simulink model "Two_area_system_with_wind_farm-DESKTOP-8DA4B7M"  (R2020a)
settings: Solver=ode23tb  StartTime=0.0  StopTime=20  RelTol=1e-3
InitFcn:
  | initAll
values from neighbouring files (symbols this model uses):
  DCgridinit = nDCgrid_init(resultsdc,wB)    [initAll.m]
  Geninit = Generator_init(opdata,SynMach_in_gidx)    [initAll.m]
  SdcgridB = resultsdc.baseMVAdc    [initAll.m]
  SgridB = resultsac.baseMVA    [initAll.m]
  VSCinit = converter_init(resultsac,resultsdc)    [initAll.m]
  wB = 2*pi*fB    (= 314.159265359)    [initAll.m]
undefined symbols (not defined in the file or in its folder): ACgirdinit, AVm0, c1, c2, c3, c4, c5, c6, cp_nom, lambda_nom, P_wind_base, Pelec_base, Pnom, Windinit
libraries: powerlib_meascontrol x9, simulink_extras x1
(part 1 of 4)
settings Model: Creator=LinSiQi  LastModifiedBy=Qiufan_Yang
settings DataIOCC: SaveOutput=off  SignalLogging=off  DSMLogging=off  SaveTime=off  ReturnWorkspaceOutputs=off
settings DebuggingCC: ArithmeticOperatorsInVariantConditions=warning
settings SFSimCC: CustomCodeUndefinedFunction=UseInterfaceOnly
settings CodeAppCC: StateflowObjectComments=on
settings SimscapeCC: SimscapeNormalizeSystem=off

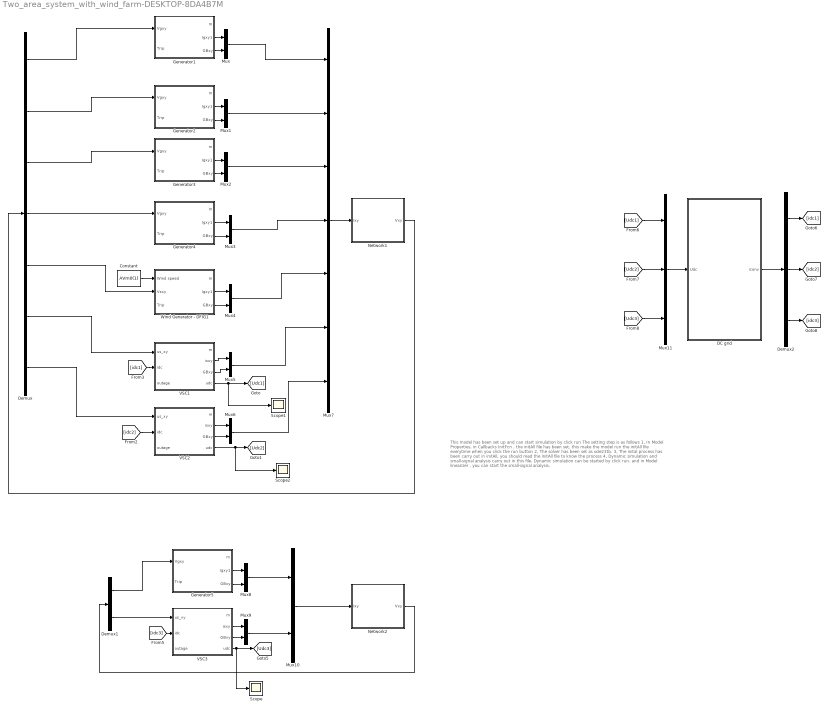
== system Two_area_system_with_wind_farm-DESKTOP-8DA4B7M ==
  note: This model has been set up and can start simulation by click run
      |
      | The setting step is as follows
      | 1, In Model Properties, in Callbacks InitFcn , the initAll file has been set, this make the model run the initAll file everytime when you click the run button
      |
      | 2, The solver has been set as ode23tb.
      |
      | 3, The inital process has been carry out in initAll, you should read the initAll file to know the process
      |
      | 4, Dynamic simulation and small-signal analysis carry out in this file. Dynamic simulation can be started by click run. and in Model linearizer , you can start the small-signal analysis.
  Constant : Constant  Value=AVm0(1)
  DC grid : Subsystem  mask{Rdc=DCgridinit.RdcA, Ldc=DCgridinit.LdcA, TDC=DCgridinit.TDC, TDCt=DCgridinit.TDCt, Idc=DCgridinit.IdcA}
  Demux : Demux  Outputs=7
  Demux1 : Demux  Outputs=2
  Demux2 : Demux  Outputs=3
  Generator1 : Subsystem  mask{wB=wB, SgenB=Geninit.SgenB(1), SgridB=SgridB, Xq=Geninit.Xq(1), Xq1=Geninit.Xq1(1), Xq11=Geninit.Xq11(1), Tq0=Geninit.Tq0(1), Tq10=Geninit.Tq10(1), Eq10=Geninit.Eq1(1), Eq110=Geninit.Eq11(1), Xd=Geninit.Xd(1), Xd1=Geninit.Xd1(1), Xd11=Geninit.Xd11(1), Td0=Geninit.Td0(1), Td10=Geninit.Td10(1), Ed10=Geninit.Ed1(1), Ed110=Geninit.Ed11(1), H=Geninit.Tj(1), D=Geninit.D(1), delta0=Geninit.Delta(1), w0=1, Pm0=Geninit.Pm0(1), Ka=Geninit.Ka(1), Tb=Geninit.Tb(1), Tc=Geninit.Tc(1), Efmin=Geninit.Efmin(1), Efmax=Geninit.Efmax(1), Vref=Geninit.Vref(1), Ef10=Geninit.Vf1(1), S_PSS=Geninit.EnablePSS(1), Kpss=Geninit.kpss(1), Tw_P=Geninit.Tw_P(1), T1_P=Geninit.T1_P(1), T2_P=Geninit.T2_P(1), T3_P=Geninit.T3_P(1), T4_P=Geninit.T4_P(1), Upmax=Geninit.Upmax(1), Upmin=Geninit.Upmin(1), S_Gov=Geninit.Enablegov(1), R=Geninit.R_G(1), Ts_G=Geninit.Ts_G(1), Tc_G=Geninit.Tc_G(1), T3_G=Geninit.T3_G(1), T4_G=Geninit.T4_G(1), T5_G=Geninit.T5_G(1), dPmax=Geninit.dPmax(1), dPmin=Geninit.dPmin(1)}
      mask prompts: S_PSS "Enable PSS"; Tw_P "Tw"; T1_P "T1"; T2_P "T2"; T3_P "T3"; T4_P "T4"; S_Gov "Enable Governor"; Ts_G "Ts"; Tc_G "Tc"; T3_G "T3"; T4_G "T4"; T5_G "T5"
      mask help: This is a six-order synchronous generator with exciter system, governor and PSS.
      mask DialogControl Container6 Prompt: Machine parameter
      mask DialogControl Container25 Prompt: Base value
      mask DialogControl Container3 Prompt: q axis parameter
      mask DialogControl ParameterGroupVar Prompt: d axis parameter
      mask DialogControl Container4 Prompt: machine parameter
      mask DialogControl Container12 Prompt: Excitation System parameter
      mask DialogControl Container22 Prompt: parameter
      mask DialogControl Container23 Prompt: inital value
      mask DialogControl Container10 Prompt: PSS parameter
      mask DialogControl Container13 Prompt: Governor parameter
  Generator2 : Subsystem  mask{wB=wB, SgenB=Geninit.SgenB(2), SgridB=SgridB, Xq=Geninit.Xq(2), Xq1=Geninit.Xq1(2), Xq11=Geninit.Xq11(2), Tq0=Geninit.Tq0(2), Tq10=Geninit.Tq10(2), Eq10=Geninit.Eq1(2), Eq110=Geninit.Eq11(2), Xd=Geninit.Xd(2), Xd1=Geninit.Xd1(2), Xd11=Geninit.Xd11(2), Td0=Geninit.Td0(2), Td10=Geninit.Td10(2), Ed10=Geninit.Ed1(2), Ed110=Geninit.Ed11(2), H=Geninit.Tj(2), D=Geninit.D(2), delta0=Geninit.Delta(2), w0=1, Pm0=Geninit.Pm0(2), Ka=Geninit.Ka(2), Tb=Geninit.Tb(2), Tc=Geninit.Tc(2), Efmin=Geninit.Efmin(2), Efmax=Geninit.Efmax(2), Vref=Geninit.Vref(2), Ef10=Geninit.Vf1(2), S_PSS=Geninit.EnablePSS(2), Kpss=Geninit.kpss(2), Tw_P=Geninit.Tw_P(2), T1_P=Geninit.T1_P(2), T2_P=Geninit.T2_P(2), T3_P=Geninit.T3_P(2), T4_P=Geninit.T4_P(2), Upmax=Geninit.Upmax(2), Upmin=Geninit.Upmin(2), S_Gov=Geninit.Enablegov(2), R=Geninit.R_G(2), Ts_G=Geninit.Ts_G(2), Tc_G=Geninit.Tc_G(2), T3_G=Geninit.T3_G(2), T4_G=Geninit.T4_G(2), T5_G=Geninit.T5_G(2), dPmax=Geninit.dPmax(2), dPmin=Geninit.dPmin(2)}
      mask prompts: S_PSS "Enable PSS"; Tw_P "Tw"; T1_P "T1"; T2_P "T2"; T3_P "T3"; T4_P "T4"; S_Gov "Enable Governor"; Ts_G "Ts"; Tc_G "Tc"; T3_G "T3"; T4_G "T4"; T5_G "T5"
      mask help: This is a six-order synchronous generator with exciter system, governor and PSS.
      mask DialogControl Container6 Prompt: Machine parameter
      mask DialogControl Container25 Prompt: Base value
      mask DialogControl Container3 Prompt: q axis parameter
      mask DialogControl ParameterGroupVar Prompt: d axis parameter
      mask DialogControl Container4 Prompt: machine parameter
      mask DialogControl Container12 Prompt: Excitation System parameter
      mask DialogControl Container22 Prompt: parameter
      mask DialogControl Container23 Prompt: inital value
      mask DialogControl Container10 Prompt: PSS parameter
      mask DialogControl Container13 Prompt: Governor parameter
  Generator3 : Subsystem  mask{wB=wB, SgenB=Geninit.SgenB(3), SgridB=SgridB, Xq=Geninit.Xq(3), Xq1=Geninit.Xq1(3), Xq11=Geninit.Xq11(3), Tq0=Geninit.Tq0(3), Tq10=Geninit.Tq10(3), Eq10=Geninit.Eq1(3), Eq110=Geninit.Eq11(3), Xd=Geninit.Xd(3), Xd1=Geninit.Xd1(3), Xd11=Geninit.Xd11(3), Td0=Geninit.Td0(3), Td10=Geninit.Td10(3), Ed10=Geninit.Ed1(3), Ed110=Geninit.Ed11(3), H=Geninit.Tj(3), D=Geninit.D(3), delta0=Geninit.Delta(3), w0=1, Pm0=Geninit.Pm0(3), Ka=Geninit.Ka(3), Tb=Geninit.Tb(3), Tc=Geninit.Tc(3), Efmin=Geninit.Efmin(3), Efmax=Geninit.Efmax(3), Vref=Geninit.Vref(3), Ef10=Geninit.Vf1(3), S_PSS=Geninit.EnablePSS(3), Kpss=Geninit.kpss(3), Tw_P=Geninit.Tw_P(3), T1_P=Geninit.T1_P(3), T2_P=Geninit.T2_P(3), T3_P=Geninit.T3_P(3), T4_P=Geninit.T4_P(3), Upmax=Geninit.Upmax(3), Upmin=Geninit.Upmin(3), S_Gov=Geninit.Enablegov(3), R=Geninit.R_G(3), Ts_G=Geninit.Ts_G(3), Tc_G=Geninit.Tc_G(3), T3_G=Geninit.T3_G(3), T4_G=Geninit.T4_G(3), T5_G=Geninit.T5_G(3), dPmax=Geninit.dPmax(3), dPmin=Geninit.dPmin(3)}
      mask prompts: S_PSS "Enable PSS"; Tw_P "Tw"; T1_P "T1"; T2_P "T2"; T3_P "T3"; T4_P "T4"; S_Gov "Enable Governor"; Ts_G "Ts"; Tc_G "Tc"; T3_G "T3"; T4_G "T4"; T5_G "T5"
      mask help: This is a six-order synchronous generator with exciter system, governor and PSS.
      mask DialogControl Container6 Prompt: Machine parameter
      mask DialogControl Container25 Prompt: Base value
      mask DialogControl Container3 Prompt: q axis parameter
      mask DialogControl ParameterGroupVar Prompt: d axis parameter
      mask DialogControl Container4 Prompt: machine parameter
      mask DialogControl Container12 Prompt: Excitation System parameter
      mask DialogControl Container22 Prompt: parameter
      mask DialogControl Container23 Prompt: inital value
      mask DialogControl Container10 Prompt: PSS parameter
      mask DialogControl Container13 Prompt: Governor parameter
  Generator4 : Subsystem  mask{wB=wB, SgenB=Geninit.SgenB(4), SgridB=SgridB, Xq=Geninit.Xq(4), Xq1=Geninit.Xq1(4), Xq11=Geninit.Xq11(4), Tq0=Geninit.Tq0(4), Tq10=Geninit.Tq10(4), Eq10=Geninit.Eq1(4), Eq110=Geninit.Eq11(4), Xd=Geninit.Xd(4), Xd1=Geninit.Xd1(4), Xd11=Geninit.Xd11(4), Td0=Geninit.Td0(4), Td10=Geninit.Td10(4), Ed10=Geninit.Ed1(4), Ed110=Geninit.Ed11(4), H=Geninit.Tj(4), D=Geninit.D(4), delta0=Geninit.Delta(4), w0=1, Pm0=Geninit.Pm0(4), Ka=Geninit.Ka(4), Tb=Geninit.Tb(4), Tc=Geninit.Tc(4), Efmin=Geninit.Efmin(4), Efmax=Geninit.Efmax(4), Vref=Geninit.Vref(4), Ef10=Geninit.Vf1(4), S_PSS=Geninit.EnablePSS(4), Kpss=Geninit.kpss(4), Tw_P=Geninit.Tw_P(4), T1_P=Geninit.T1_P(4), T2_P=Geninit.T2_P(4), T3_P=Geninit.T3_P(4), T4_P=Geninit.T4_P(4), Upmax=Geninit.Upmax(4), Upmin=Geninit.Upmin(4), S_Gov=Geninit.Enablegov(4), R=Geninit.R_G(4), Ts_G=Geninit.Ts_G(4), Tc_G=Geninit.Tc_G(4), T3_G=Geninit.T3_G(4), T4_G=Geninit.T4_G(4), T5_G=Geninit.T5_G(4), dPmax=Geninit.dPmax(4), dPmin=Geninit.dPmin(4)}
      mask prompts: S_PSS "Enable PSS"; Tw_P "Tw"; T1_P "T1"; T2_P "T2"; T3_P "T3"; T4_P "T4"; S_Gov "Enable Governor"; Ts_G "Ts"; Tc_G "Tc"; T3_G "T3"; T4_G "T4"; T5_G "T5"
      mask help: This is a six-order synchronous generator with exciter system, governor and PSS.
      mask DialogControl Container6 Prompt: Machine parameter
      mask DialogControl Container25 Prompt: Base value
      mask DialogControl Container3 Prompt: q axis parameter
      mask DialogControl ParameterGroupVar Prompt: d axis parameter
      mask DialogControl Container4 Prompt: machine parameter
      mask DialogControl Container12 Prompt: Excitation System parameter
      mask DialogControl Container22 Prompt: parameter
      mask DialogControl Container23 Prompt: inital value
      mask DialogControl Container10 Prompt: PSS parameter
      mask DialogControl Container13 Prompt: Governor parameter
  Generator5 : Subsystem  mask{wB=wB, SgenB=Geninit.SgenB(5), SgridB=SgridB, Xq=Geninit.Xq(5), Xq1=Geninit.Xq1(5), Xq11=Geninit.Xq11(5), Tq0=Geninit.Tq0(5), Tq10=Geninit.Tq10(5), Eq10=Geninit.Eq1(5), Eq110=Geninit.Eq11(5), Xd=Geninit.Xd(5), Xd1=Geninit.Xd1(5), Xd11=Geninit.Xd11(5), Td0=Geninit.Td0(5), Td10=Geninit.Td10(5), Ed10=Geninit.Ed1(5), Ed110=Geninit.Ed11(5), H=Geninit.Tj(5), D=Geninit.D(5), delta0=Geninit.Delta(5), w0=1, Pm0=Geninit.Pm0(5), Ka=Geninit.Ka(5), Tb=Geninit.Tb(5), Tc=Geninit.Tc(5), Efmin=Geninit.Efmin(5), Efmax=Geninit.Efmax(5), Vref=Geninit.Vref(5), Ef10=Geninit.Vf1(5), S_PSS=Geninit.EnablePSS(5), Kpss=Geninit.kpss(5), Tw_P=Geninit.Tw_P(5), T1_P=Geninit.T1_P(5), T2_P=Geninit.T2_P(5), T3_P=Geninit.T3_P(5), T4_P=Geninit.T4_P(5), Upmax=Geninit.Upmax(5), Upmin=Geninit.Upmin(5), S_Gov=Geninit.Enablegov(5), R=Geninit.R_G(5), Ts_G=Geninit.Ts_G(5), Tc_G=Geninit.Tc_G(5), T3_G=Geninit.T3_G(5), T4_G=Geninit.T4_G(5), T5_G=Geninit.T5_G(5), dPmax=Geninit.dPmax(5), dPmin=Geninit.dPmin(5)}
      mask prompts: S_PSS "Enable PSS"; Tw_P "Tw"; T1_P "T1"; T2_P "T2"; T3_P "T3"; T4_P "T4"; S_Gov "Enable Governor"; Ts_G "Ts"; Tc_G "Tc"; T3_G "T3"; T4_G "T4"; T5_G "T5"
      mask help: This is a six-order synchronous generator with exciter system, governor and PSS.
      mask DialogControl Container6 Prompt: Machine parameter
      mask DialogControl Container25 Prompt: Base value
      mask DialogControl Container3 Prompt: q axis parameter
      mask DialogControl ParameterGroupVar Prompt: d axis parameter
      mask DialogControl Container4 Prompt: machine parameter
      mask DialogControl Container12 Prompt: Excitation System parameter
      mask DialogControl Container22 Prompt: parameter
      mask DialogControl Container23 Prompt: inital value
      mask DialogControl Container10 Prompt: PSS parameter
      mask DialogControl Container13 Prompt: Governor parameter
  Mux{,1..6,8..10} (10 alike) : Mux  Inputs=2
  Mux11 : Mux  Inputs=3
  Mux7 : Mux  Inputs=7
  Network1 : Subsystem  mask{busdata=ACgirdinit.busdata{1}, linedata=ACgirdinit.linedata{1}, VSS0=ACgirdinit.VSS0{1}, LINE=ACgirdinit.fline{1}, fbus=ACgirdinit.FBUS(1), ng=ACgirdinit.ng{1}, Currentin_idx=ACgirdinit.Currentin_idx{1}}
  Network2 : Subsystem  mask{busdata=ACgirdinit.busdata{2}, linedata=ACgirdinit.linedata{2}, VSS0=ACgirdinit.VSS0{2}, LINE=ACgirdinit.fline{2}, fbus=ACgirdinit.FBUS(2), ng=ACgirdinit.ng{2}, Currentin_idx=ACgirdinit.Currentin_idx{2}}
  Scope : Scope
  Scope1 : Scope
  Scope2 : Scope
  VSC1 : Subsystem  mask{Vdcbase=VSCinit.Vdcbase(1), Vnom=VSCinit.Vacbase(1), SvscB=VSCinit.SvscBi(1), SgridB=SgridB, SdcgridB=SdcgridB, Kppll_VSC=VSCinit.Kppll(1), Kipll_VSC=VSCinit.Kipll(1), Dels_hvdc=VSCinit.Dels_hvdc(1), CeqA=VSCinit.CeqA(1), UeqA=VSCinit.UeqA(1), Lpr=VSCinit.Lpr(1), Rpr=VSCinit.Rpr(1), wB=wB, Is_xA_0=VSCinit.Isx0(1), Is_yA_0=VSCinit.Isy0(1), d_axis_control=VSCinit.d_axis_control(1), KpP_VSC_A=VSCinit.KpP(1), KiP_VSC_A=VSCinit.KiP(1), Kpdc_VSC_A=VSCinit.Kpdc(1), Kidc_VSC_A=VSCinit.Kidc(1), KpId_VSC_A=VSCinit.KpId(1), KiId_VSC_A=VSCinit.KiId(1), q_axis_control=VSCinit.q_axis_control(1), KpQ_VSC_A=VSCinit.KpQ(1), KiQ_VSC_A=VSCinit.KiQ(1), Kpac_VSC_A=VSCinit.Kpac(1), Kiac_VSC_A=VSCinit.Kiac(1), KpIq_VSC_A=VSCinit.KpIq(1), KiIq_VSC_A=VSCinit.KiIq(1), Md_A_0=VSCinit.Md0(1), Mq_A_0=VSCinit.Mq0(1), Nd_A_0=VSCinit.Nd0(1), Nq_A_0=VSCinit.Nq0(1), Pref=VSCinit.Pref(1), Udcref=VSCinit.Udcref(1), Qref=VSCinit.Qref(1), Uref=VSCinit.Uref(1)}
      mask prompts: Vnom "Vacbase"; Kppll_VSC "Kppll"; Kipll_VSC "Kipll"; KpP_VSC_A "KpP"; KiP_VSC_A "KiP"; Kpdc_VSC_A "Kpdc"; Kidc_VSC_A "Kidc"; KpId_VSC_A "KpId"; KiId_VSC_A "KiId"; KpQ_VSC_A "KpQ"; KiQ_VSC_A "KiQ"; Kpac_VSC_A "Kpac"; Kiac_VSC_A "Kiac"; KpIq_VSC_A "KpIq"; KiIq_VSC_A "KiIq"
      mask DialogControl Container48 Prompt: Base value
      mask DialogControl Container7 Prompt: PLL
      mask DialogControl Container5 Prompt: Control parameter
      mask DialogControl Container8 Prompt: inital value
      mask DialogControl Container12 Prompt: DC side
      mask DialogControl Container13 Prompt: Parameter
      mask DialogControl Container15 Prompt: Initial value
      mask DialogControl Container9 Prompt: AC side
      mask DialogControl Container10 Prompt: Parameter
      mask DialogControl Container11 Prompt: Initial value
      mask DialogControl Container18 Prompt: Control parameter
      mask DialogControl Container19 Prompt: d_axis_control parameter
      mask DialogControl Container23 Prompt: d_axis_control=1
      mask DialogControl Container24 Prompt: d_axis_control=2
      mask DialogControl Container26 Prompt: inner current control
      mask DialogControl Container21 Prompt: q_axis_control parameter
      mask DialogControl Container29 Prompt: q_axis_control=1
      mask DialogControl Container30 Prompt: q_axis_control=2
      mask DialogControl Container31 Prompt: inner current control
      mask DialogControl Container22 Prompt: inital value
      mask DialogControl Container35 Prompt: outer controller
      mask DialogControl Container36 Prompt: inner control
      mask DialogControl Container38 Prompt: Reference
  VSC2 : Subsystem  mask{Vdcbase=VSCinit.Vdcbase(2), Vnom=VSCinit.Vacbase(2), SvscB=VSCinit.SvscBi(2), SgridB=SgridB, SdcgridB=SdcgridB, Kppll_VSC=VSCinit.Kppll(2), Kipll_VSC=VSCinit.Kipll(2), Dels_hvdc=VSCinit.Dels_hvdc(2), CeqA=VSCinit.CeqA(2), UeqA=VSCinit.UeqA(2), Lpr=VSCinit.Lpr(2), Rpr=VSCinit.Rpr(2), wB=wB, Is_xA_0=VSCinit.Isx0(2), Is_yA_0=VSCinit.Isy0(2), d_axis_control=VSCinit.d_axis_control(2), KpP_VSC_A=VSCinit.KpP(2), KiP_VSC_A=VSCinit.KiP(2), Kpdc_VSC_A=VSCinit.Kpdc(2), Kidc_VSC_A=VSCinit.Kidc(2), KpId_VSC_A=VSCinit.KpId(2), KiId_VSC_A=VSCinit.KiId(2), q_axis_control=VSCinit.q_axis_control(2), KpQ_VSC_A=VSCinit.KpQ(2), KiQ_VSC_A=VSCinit.KiQ(2), Kpac_VSC_A=VSCinit.Kpac(2), Kiac_VSC_A=VSCinit.Kiac(2), KpIq_VSC_A=VSCinit.KpIq(2), KiIq_VSC_A=VSCinit.KiIq(2), Md_A_0=VSCinit.Md0(2), Mq_A_0=VSCinit.Mq0(2), Nd_A_0=VSCinit.Nd0(2), Nq_A_0=VSCinit.Nq0(2), Pref=VSCinit.Pref(2), Udcref=VSCinit.Udcref(2), Qref=VSCinit.Qref(2), Uref=VSCinit.Uref(2)}
      mask prompts: Vnom "Vacbase"; Kppll_VSC "Kppll"; Kipll_VSC "Kipll"; KpP_VSC_A "KpP"; KiP_VSC_A "KiP"; Kpdc_VSC_A "Kpdc"; Kidc_VSC_A "Kidc"; KpId_VSC_A "KpId"; KiId_VSC_A "KiId"; KpQ_VSC_A "KpQ"; KiQ_VSC_A "KiQ"; Kpac_VSC_A "Kpac"; Kiac_VSC_A "Kiac"; KpIq_VSC_A "KpIq"; KiIq_VSC_A "KiIq"
      mask DialogControl Container48 Prompt: Base value
      mask DialogControl Container7 Prompt: PLL
      mask DialogControl Container5 Prompt: Control parameter
      mask DialogControl Container8 Prompt: inital value
      mask DialogControl Container12 Prompt: DC side
      mask DialogControl Container13 Prompt: Parameter
      mask DialogControl Container15 Prompt: Initial value
      mask DialogControl Container9 Prompt: AC side
      mask DialogControl Container10 Prompt: Parameter
      mask DialogControl Container11 Prompt: Initial value
      mask DialogControl Container18 Prompt: Control parameter
      mask DialogControl Container19 Prompt: d_axis_control parameter
      mask DialogControl Container23 Prompt: d_axis_control=1
      mask DialogControl Container24 Prompt: d_axis_control=2
      mask DialogControl Container26 Prompt: inner current control
      mask DialogControl Container21 Prompt: q_axis_control parameter
      mask DialogControl Container29 Prompt: q_axis_control=1
      mask DialogControl Container30 Prompt: q_axis_control=2
      mask DialogControl Container31 Prompt: inner current control
      mask DialogControl Container22 Prompt: inital value
      mask DialogControl Container35 Prompt: outer controller
      mask DialogControl Container36 Prompt: inner control
      mask DialogControl Container38 Prompt: Reference
  VSC3 : Subsystem  mask{Vdcbase=VSCinit.Vdcbase(3), Vnom=VSCinit.Vacbase(3), SvscB=VSCinit.SvscBi(3), SgridB=SgridB, SdcgridB=SdcgridB, Kppll_VSC=VSCinit.Kppll(3), Kipll_VSC=VSCinit.Kipll(3), Dels_hvdc=VSCinit.Dels_hvdc(3), CeqA=VSCinit.CeqA(3), UeqA=VSCinit.UeqA(3), Lpr=VSCinit.Lpr(3), Rpr=VSCinit.Rpr(3), wB=wB, Is_xA_0=VSCinit.Isx0(3), Is_yA_0=VSCinit.Isy0(3), d_axis_control=VSCinit.d_axis_control(3), KpP_VSC_A=VSCinit.KpP(3), KiP_VSC_A=VSCinit.KiP(3), Kpdc_VSC_A=VSCinit.Kpdc(3), Kidc_VSC_A=VSCinit.Kidc(3), KpId_VSC_A=VSCinit.KpId(3), KiId_VSC_A=VSCinit.KiId(3), q_axis_control=VSCinit.q_axis_control(3), KpQ_VSC_A=VSCinit.KpQ(3), KiQ_VSC_A=VSCinit.KiQ(3), Kpac_VSC_A=VSCinit.Kpac(3), Kiac_VSC_A=VSCinit.Kiac(3), KpIq_VSC_A=VSCinit.KpIq(3), KiIq_VSC_A=VSCinit.KiIq(3), Md_A_0=VSCinit.Md0(3), Mq_A_0=VSCinit.Mq0(3), Nd_A_0=VSCinit.Nd0(3), Nq_A_0=VSCinit.Nq0(3), Pref=VSCinit.Pref(3), Udcref=VSCinit.Udcref(3), Qref=VSCinit.Qref(3), Uref=VSCinit.Uref(3)}
      mask prompts: Vnom "Vacbase"; Kppll_VSC "Kppll"; Kipll_VSC "Kipll"; KpP_VSC_A "KpP"; KiP_VSC_A "KiP"; Kpdc_VSC_A "Kpdc"; Kidc_VSC_A "Kidc"; KpId_VSC_A "KpId"; KiId_VSC_A "KiId"; KpQ_VSC_A "KpQ"; KiQ_VSC_A "KiQ"; Kpac_VSC_A "Kpac"; Kiac_VSC_A "Kiac"; KpIq_VSC_A "KpIq"; KiIq_VSC_A "KiIq"
      mask DialogControl Container48 Prompt: Base value
      mask DialogControl Container7 Prompt: PLL
      mask DialogControl Container5 Prompt: Control parameter
      mask DialogControl Container8 Prompt: inital value
      mask DialogControl Container12 Prompt: DC side
      mask DialogControl Container13 Prompt: Parameter
      mask DialogControl Container15 Prompt: Initial value
      mask DialogControl Container9 Prompt: AC side
      mask DialogControl Container10 Prompt: Parameter
      mask DialogControl Container11 Prompt: Initial value
      mask DialogControl Container18 Prompt: Control parameter
      mask DialogControl Container19 Prompt: d_axis_control parameter
      mask DialogControl Container23 Prompt: d_axis_control=1
      mask DialogControl Container24 Prompt: d_axis_control=2
      mask DialogControl Container26 Prompt: inner current control
      mask DialogControl Container21 Prompt: q_axis_control parameter
      mask DialogControl Container29 Prompt: q_axis_control=1
      mask DialogControl Container30 Prompt: q_axis_control=2
      mask DialogControl Container31 Prompt: inner current control
      mask DialogControl Container22 Prompt: inital value
      mask DialogControl Container35 Prompt: outer controller
      mask DialogControl Container36 Prompt: inner control
      mask DialogControl Container38 Prompt: Reference
  Wind Generator - DFIG1 : Subsystem  mask{NN=Windinit.NN(1), SwgBi=Windinit.SwgBi(1), SmecBi=100, SgridB=SgridB, Atheta=Windinit.Atheta(1), Kppll=Windinit.Kppll_wind(1), Kipll=Windinit.Kipll_wind(1), pitch=[500 45 2], Srotors=1.3, H=Windinit.H(1), Wr0=Windinit.Wr0(1), Xa=Windinit.Xa(1), Xa1=Windinit.Xa1(1), Lm=Windinit.Lm(1), Lr=Windinit.Lr(1), Rs=Windinit.Rs(1), Ls=Windinit.Ls(1), Ta0=Windinit.Ta0(1), NPf=Windinit.NPf(1), Za=Windinit.Za{1}, Ex0=Windinit.Ex_ref(1), Ey0=Windinit.Ey_ref(1), wB=wB, KpP_rw=Windinit.KpP_rw(1), KiP_rw=Windinit.KiP_rw(1), KpId_rw=Windinit.KpId_rw(1), KiId_rw=Windinit.KiId_rw(1), KpQ_rw=Windinit.KpQ_rw(1), KiQ_rw=Windinit.KiQ_rw(1), KpIq_rw=Windinit.KpIq_rw(1), KiIq_rw=Windinit.KiIq_rw(1), Ird_ref=Windinit.Ird_ref(1), Irq_ref=Windinit.Irq_ref(1), Qs0=Windinit.Qs0(1), KpDC_gw=Windinit.KpDC_gw(1), KiDC_gw=Windinit.KiDC_gw(1), KpId_gw=Windinit.KpId_gw(1), KiId_gw=Windinit.KiId_gw(1), KpIq_gw=Windinit.KpIq_gw(1), KiIq_gw=Windinit.KiIq_gw(1), Vdc_w=Windinit.Vdc_w(1), Icd_ref=Windinit.Icd_ref(1), Icq_ref=Windinit.Icq_ref(1), Vcd_ref=Windinit.Vcd_ref(1), Vcq_ref=Windinit.Vcq_ref(1), Lg=Windinit.Lg(1), Rg=Windinit.Rg(1), Icx0=Windinit.Icx0(1), Icy0=Windinit.Icy0(1), C_w=Windinit.C_w(1), Vdc0=Windinit.Vdc0(1)}
      mask prompts: pitch "pitch_gain，pitch_max，pitch_rate"; Srotors "Start Rotor Speed"; Ex0 "Ex"; Ey0 "Ey"
      mask init:
      | pitch_gain=pitch(1);
      | pitch_max=pitch(2);
      | pitch_rate=pitch(3);
      | 
      | %该风机模型的基准容量
      | 
      | SwgeqB=SwgBi.*NN;
      mask DialogControl Container4 Prompt: PLL/Wind turbine
      mask DialogControl Container31 Prompt: Base value
      mask DialogControl Container23 Prompt: PLL
      mask DialogControl Container6 Prompt: inital value
      mask DialogControl Container5 Prompt: PI parameter
      mask DialogControl Container24 Prompt: Wind turbine
      mask DialogControl Container25 Prompt: pitch control
      mask DialogControl Container7 Prompt: Machine parameter
      mask DialogControl Container8 Prompt: Rotor
      mask DialogControl Container9 Prompt: Machine
      mask DialogControl Container10 Prompt: parameter
      mask DialogControl Container11 Prompt: inital value
      mask DialogControl Container12 Prompt: Rotor side control
      mask DialogControl Container13 Prompt: Control parameter
      mask DialogControl Container14 Prompt: Initial value
      mask DialogControl Container15 Prompt: reactive power
      mask DialogControl Container16 Prompt: Grid side control
      mask DialogControl Container17 Prompt: parameter
      mask DialogControl Container18 Prompt: reference
      mask DialogControl Container19 Prompt: inital value
      mask DialogControl Container20 Prompt: converter function
      mask DialogControl Container21 Prompt: inital value
      mask DialogControl Container22 Prompt: DC function
  wires:
  Generator1/2(Igxy1) -> Mux/1
  Generator1/3(GBxy) -> Mux/2
  Generator2/2(Igxy1) -> Mux1/1
  Generator2/3(GBxy) -> Mux1/2
  Generator3/2(Igxy1) -> Mux2/1
  Generator3/3(GBxy) -> Mux2/2
  Generator4/2(Igxy1) -> Mux3/1
  Generator4/3(GBxy) -> Mux3/2
  Wind Generator - DFIG1/2(Igxy1) -> Mux4/1
  Wind Generator - DFIG1/3(GBxy) -> Mux4/2
  VSC1/2(isxy) -> Mux5/1
  VSC1/3(GBxy) -> Mux5/2
  VSC2/2(isxy) -> Mux6/1
  VSC2/3(GBxy) -> Mux6/2
  Mux7/1 -> Network1/1(Ixy)
  Mux/1 -> Mux7/1
  Mux1/1 -> Mux7/2
  Mux2/1 -> Mux7/3
  Mux3/1 -> Mux7/4
  Mux4/1 -> Mux7/5
  Mux5/1 -> Mux7/6
  Mux6/1 -> Mux7/7
  Network1/1(Vxy) -> Demux/1
  Demux/1 -> Generator1/1(Vgxy)
  Demux/2 -> Generator2/1(Vgxy)
  Demux/3 -> Generator3/1(Vgxy)
  Demux/4 -> Generator4/1(Vgxy)
  Demux/5 -> Wind Generator - DFIG1/2(Vsxy)
  Demux/6 -> VSC1/1(us_xy)
  Demux/7 -> VSC2/1(us_xy)
  Constant/1 -> Wind Generator - DFIG1/1(Wind speed)
  VSC1/4(udc) -> Scope1/1, [Udc1]
  VSC2/4(udc) -> Scope2/1, [Udc2]
  [idc2] -> VSC2/2(idc)
  [idc1] -> VSC1/2(idc)
  Generator5/2(Igxy1) -> Mux8/1
  Generator5/3(GBxy) -> Mux8/2
  VSC3/2(isxy) -> Mux9/1
  VSC3/3(GBxy) -> Mux9/2
  Mux9/1 -> Mux10/2
  Mux8/1 -> Mux10/1
  Mux10/1 -> Network2/1(Ixy)
  Demux1/1 -> Generator5/1(Vgxy)
  Demux1/2 -> VSC3/1(us_xy)
  [idc3] -> VSC3/2(idc)
  VSC3/4(udc) -> Scope/1, [Udc3]
  Network2/1(Vxy) -> Demux1/1
  [Udc1] -> Mux11/1
  [Udc2] -> Mux11/2
  [Udc3] -> Mux11/3
  Mux11/1 -> DC grid/1(Udc)
  DC grid/1(iconv) -> Demux2/1
  Demux2/1 -> [idc1]
  Demux2/2 -> [idc2]
  Demux2/3 -> [idc3]

== system Two_area_system_with_wind_farm-DESKTOP-8DA4B7M/DC grid ==
  Udc : Inport
  Gain : Gain  Gain=TDCt  Multiplication=Matrix(K*u) (u vector)
  Gain1 : Gain  Gain=TDC  Multiplication=Matrix(K*u) (u vector)
  Idc_line : Integrator  InitialCondition=Idc
  K6 : Gain  Gain=Ldc  SaturateOnIntegerOverflow=on  OutDataTypeStr=Inherit: Same as input  ParamDataTypeStr=Inherit: Same as input
  K7 : Gain  Gain=Rdc  SaturateOnIntegerOverflow=on  OutDataTypeStr=Inherit: Same as input  ParamDataTypeStr=Inherit: Same as input
  Sum1 : Sum  Inputs=|+-  SaturateOnIntegerOverflow=on
  iconv : Outport
  wires:
  K6/1 -> Idc_line/1
  Idc_line/1 -> Gain1/1, K7/1
  Sum1/1 -> K6/1
  K7/1 -> Sum1/2
  Udc/1 -> Gain/1
  Gain/1 -> Sum1/1
  Gain1/1 -> iconv/1

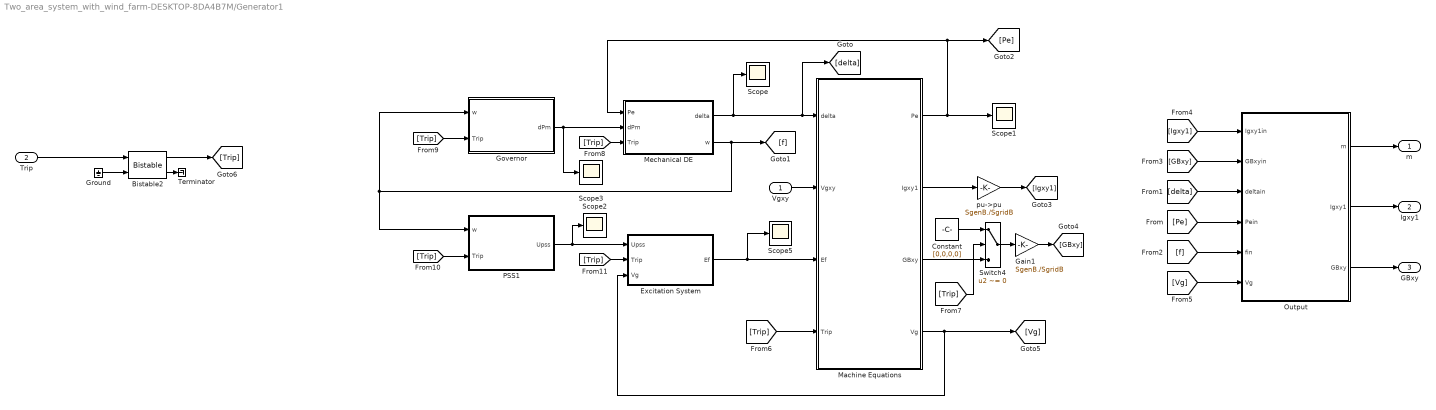
== system Two_area_system_with_wind_farm-DESKTOP-8DA4B7M/Generator1 ==
  Vgxy : Inport
  Trip : Inport  Port=2
  Bistable2 : powerlib_meascontrol/Logic/Bistable  Qpriority=Set  ic=0  Ts=0
      settings: SourceProductBaseCode=PS
  Constant : Constant  Value=[0,0,0,0]
  Excitation System : Subsystem
  Gain1 : Gain  Gain=SgenB./SgridB
  Governor : Subsystem
  Ground : Ground
  "Machine Equations " : Subsystem
  Mechanical DE : Subsystem
  Output : Subsystem
  PSS1 : Subsystem
  Scope{,1..3,5} (5 alike) : Scope
  Switch4 : Switch  Criteria=u2 ~= 0  Threshold=0.5  SaturateOnIntegerOverflow=on
  Terminator : Terminator
  pu->pu : Gain  Gain=SgenB./SgridB
  m : Outport
  Igxy1 : Outport  Port=2
  GBxy : Outport  Port=3
  wires:
  Gain1/1 -> [GBxy]
  pu->pu/1 -> [Igxy1]
  [Trip] -> PSS1/2(Trip)
  [Trip] -> Governor/2(Trip)
  [GBxy] -> Output/2(GBxyin)
  [Trip] -> Excitation System/2(Trip)
  Output/1(m) -> m/1
  Mechanical DE/1(delta) -> Scope/1, "Machine Equations "/1(delta), [delta]
  Bistable2/2 -> Terminator/1
  [f] -> Output/5(fin)
  Output/2(Igxy1) -> Igxy1/1
  PSS1/1(Upss) -> Excitation System/1(Upss), Scope2/1
  "Machine Equations "/3(GBxy) -> Switch4/3
  Vgxy/1 -> "Machine Equations "/2(Vgxy)
  Constant/1 -> Switch4/1
  "Machine Equations "/2(Igxy1) -> pu->pu/1
  Governor/1(dPm) -> Mechanical DE/2(dPm), Scope3/1
  [delta] -> Output/3(deltain)
  [Vg] -> Output/6(Vg)
  [Igxy1] -> Output/1(Igxy1in)
  Mechanical DE/2(w) -> Governor/1(w), PSS1/1(w), [f]
  Output/3(GBxy) -> GBxy/1
  Excitation System/1(Ef) -> Scope5/1, "Machine Equations "/3(Ef)
  "Machine Equations "/4(Vg) -> [Vg], Excitation System/3(Vg)
  [Trip] -> "Machine Equations "/4(Trip)
  [Trip] -> Switch4/2
  Bistable2/1 -> [Trip]
  "Machine Equations "/1(Pe) -> Scope1/1, Mechanical DE/1(Pe), [Pe]
  [Pe] -> Output/4(Pein)
  Switch4/1 -> Gain1/1
  Trip/1 -> Bistable2/1
  Ground/1 -> Bistable2/2
  [Trip] -> Mechanical DE/3(Trip)

== system Two_area_system_with_wind_farm-DESKTOP-8DA4B7M/Generator2 ==
  Vgxy : Inport
  Trip : Inport  Port=2
  Bistable2 : powerlib_meascontrol/Logic/Bistable  Qpriority=Set  ic=0  Ts=0
      settings: SourceProductBaseCode=PS
  Constant : Constant  Value=[0,0,0,0]
  Excitation System : Subsystem
  Gain1 : Gain  Gain=SgenB./SgridB
  Governor : Subsystem
  Ground : Ground
  "Machine Equations " : Subsystem
  Mechanical DE : Subsystem
  Output : Subsystem
  PSS1 : Subsystem
  Scope{,1..3,5} (5 alike) : Scope
  Switch4 : Switch  Criteria=u2 ~= 0  Threshold=0.5  SaturateOnIntegerOverflow=on
  Terminator : Terminator
  pu->pu : Gain  Gain=SgenB./SgridB
  m : Outport
  Igxy1 : Outport  Port=2
  GBxy : Outport  Port=3
  wires:
  Gain1/1 -> [GBxy]
  pu->pu/1 -> [Igxy1]
  [Trip] -> PSS1/2(Trip)
  [Trip] -> Governor/2(Trip)
  [GBxy] -> Output/2(GBxyin)
  [Trip] -> Excitation System/2(Trip)
  Output/1(m) -> m/1
  Mechanical DE/1(delta) -> Scope/1, "Machine Equations "/1(delta), [delta]
  Bistable2/2 -> Terminator/1
  [f] -> Output/5(fin)
  Output/2(Igxy1) -> Igxy1/1
  PSS1/1(Upss) -> Excitation System/1(Upss), Scope2/1
  "Machine Equations "/3(GBxy) -> Switch4/3
  Vgxy/1 -> "Machine Equations "/2(Vgxy)
  Constant/1 -> Switch4/1
  "Machine Equations "/2(Igxy1) -> pu->pu/1
  Governor/1(dPm) -> Mechanical DE/2(dPm), Scope3/1
  [delta] -> Output/3(deltain)
  [Vg] -> Output/6(Vg)
  [Igxy1] -> Output/1(Igxy1in)
  Mechanical DE/2(w) -> Governor/1(w), PSS1/1(w), [f]
  Output/3(GBxy) -> GBxy/1
  Excitation System/1(Ef) -> Scope5/1, "Machine Equations "/3(Ef)
  "Machine Equations "/4(Vg) -> [Vg], Excitation System/3(Vg)
  [Trip] -> "Machine Equations "/4(Trip)
  [Trip] -> Switch4/2
  Bistable2/1 -> [Trip]
  "Machine Equations "/1(Pe) -> Scope1/1, Mechanical DE/1(Pe), [Pe]
  [Pe] -> Output/4(Pein)
  Switch4/1 -> Gain1/1
  Trip/1 -> Bistable2/1
  Ground/1 -> Bistable2/2
  [Trip] -> Mechanical DE/3(Trip)

== system Two_area_system_with_wind_farm-DESKTOP-8DA4B7M/Generator3 ==
  Vgxy : Inport
  Trip : Inport  Port=2
  Bistable2 : powerlib_meascontrol/Logic/Bistable  Qpriority=Set  ic=0  Ts=0
      settings: SourceProductBaseCode=PS
  Constant : Constant  Value=[0,0,0,0]
  Excitation System : Subsystem
  Gain1 : Gain  Gain=SgenB./SgridB
  Governor : Subsystem
  Ground : Ground
  "Machine Equations " : Subsystem
  Mechanical DE : Subsystem
  Output : Subsystem
  PSS1 : Subsystem
  Scope{,1..3,5} (5 alike) : Scope
  Switch4 : Switch  Criteria=u2 ~= 0  Threshold=0.5  SaturateOnIntegerOverflow=on
  Terminator : Terminator
  pu->pu : Gain  Gain=SgenB./SgridB
  m : Outport
  Igxy1 : Outport  Port=2
  GBxy : Outport  Port=3
  wires:
  Gain1/1 -> [GBxy]
  pu->pu/1 -> [Igxy1]
  [Trip] -> PSS1/2(Trip)
  [Trip] -> Governor/2(Trip)
  [GBxy] -> Output/2(GBxyin)
  [Trip] -> Excitation System/2(Trip)
  Output/1(m) -> m/1
  Mechanical DE/1(delta) -> Scope/1, "Machine Equations "/1(delta), [delta]
  Bistable2/2 -> Terminator/1
  [f] -> Output/5(fin)
  Output/2(Igxy1) -> Igxy1/1
  PSS1/1(Upss) -> Excitation System/1(Upss), Scope2/1
  "Machine Equations "/3(GBxy) -> Switch4/3
  Vgxy/1 -> "Machine Equations "/2(Vgxy)
  Constant/1 -> Switch4/1
  "Machine Equations "/2(Igxy1) -> pu->pu/1
  Governor/1(dPm) -> Mechanical DE/2(dPm), Scope3/1
  [delta] -> Output/3(deltain)
  [Vg] -> Output/6(Vg)
  [Igxy1] -> Output/1(Igxy1in)
  Mechanical DE/2(w) -> Governor/1(w), PSS1/1(w), [f]
  Output/3(GBxy) -> GBxy/1
  Excitation System/1(Ef) -> Scope5/1, "Machine Equations "/3(Ef)
  "Machine Equations "/4(Vg) -> [Vg], Excitation System/3(Vg)
  [Trip] -> "Machine Equations "/4(Trip)
  [Trip] -> Switch4/2
  Bistable2/1 -> [Trip]
  "Machine Equations "/1(Pe) -> Scope1/1, Mechanical DE/1(Pe), [Pe]
  [Pe] -> Output/4(Pein)
  Switch4/1 -> Gain1/1
  Trip/1 -> Bistable2/1
  Ground/1 -> Bistable2/2
  [Trip] -> Mechanical DE/3(Trip)

== system Two_area_system_with_wind_farm-DESKTOP-8DA4B7M/Generator4 ==
  Vgxy : Inport
  Trip : Inport  Port=2
  Bistable2 : powerlib_meascontrol/Logic/Bistable  Qpriority=Set  ic=0  Ts=0
      settings: SourceProductBaseCode=PS
  Constant : Constant  Value=[0,0,0,0]
  Excitation System : Subsystem
  Gain1 : Gain  Gain=SgenB./SgridB
  Governor : Subsystem
  Ground : Ground
  "Machine Equations " : Subsystem
  Mechanical DE : Subsystem
  Output : Subsystem
  PSS1 : Subsystem
  Scope{,1..3,5} (5 alike) : Scope
  Switch4 : Switch  Criteria=u2 ~= 0  Threshold=0.5  SaturateOnIntegerOverflow=on
  Terminator : Terminator
  pu->pu : Gain  Gain=SgenB./SgridB
  m : Outport
  Igxy1 : Outport  Port=2
  GBxy : Outport  Port=3
  wires:
  Gain1/1 -> [GBxy]
  pu->pu/1 -> [Igxy1]
  [Trip] -> PSS1/2(Trip)
  [Trip] -> Governor/2(Trip)
  [GBxy] -> Output/2(GBxyin)
  [Trip] -> Excitation System/2(Trip)
  Output/1(m) -> m/1
  Mechanical DE/1(delta) -> Scope/1, "Machine Equations "/1(delta), [delta]
  Bistable2/2 -> Terminator/1
  [f] -> Output/5(fin)
  Output/2(Igxy1) -> Igxy1/1
  PSS1/1(Upss) -> Excitation System/1(Upss), Scope2/1
  "Machine Equations "/3(GBxy) -> Switch4/3
  Vgxy/1 -> "Machine Equations "/2(Vgxy)
  Constant/1 -> Switch4/1
  "Machine Equations "/2(Igxy1) -> pu->pu/1
  Governor/1(dPm) -> Mechanical DE/2(dPm), Scope3/1
  [delta] -> Output/3(deltain)
  [Vg] -> Output/6(Vg)
  [Igxy1] -> Output/1(Igxy1in)
  Mechanical DE/2(w) -> Governor/1(w), PSS1/1(w), [f]
  Output/3(GBxy) -> GBxy/1
  Excitation System/1(Ef) -> Scope5/1, "Machine Equations "/3(Ef)
  "Machine Equations "/4(Vg) -> [Vg], Excitation System/3(Vg)
  [Trip] -> "Machine Equations "/4(Trip)
  [Trip] -> Switch4/2
  Bistable2/1 -> [Trip]
  "Machine Equations "/1(Pe) -> Scope1/1, Mechanical DE/1(Pe), [Pe]
  [Pe] -> Output/4(Pein)
  Switch4/1 -> Gain1/1
  Trip/1 -> Bistable2/1
  Ground/1 -> Bistable2/2
  [Trip] -> Mechanical DE/3(Trip)

== system Two_area_system_with_wind_farm-DESKTOP-8DA4B7M/Generator5 ==
  Vgxy : Inport
  Trip : Inport  Port=2
  Bistable2 : powerlib_meascontrol/Logic/Bistable  Qpriority=Set  ic=0  Ts=0
      settings: SourceProductBaseCode=PS
  Constant : Constant  Value=[0,0,0,0]
  Excitation System : Subsystem
  Gain1 : Gain  Gain=SgenB./SgridB
  Governor : Subsystem
  Ground : Ground
  "Machine Equations " : Subsystem
  Mechanical DE : Subsystem
  Output : Subsystem
  PSS1 : Subsystem
  Scope{,1..3,5} (5 alike) : Scope
  Switch4 : Switch  Criteria=u2 ~= 0  Threshold=0.5  SaturateOnIntegerOverflow=on
  Terminator : Terminator
  pu->pu : Gain  Gain=SgenB./SgridB
  m : Outport
  Igxy1 : Outport  Port=2
  GBxy : Outport  Port=3
  wires:
  Gain1/1 -> [GBxy]
  pu->pu/1 -> [Igxy1]
  [Trip] -> PSS1/2(Trip)
  [Trip] -> Governor/2(Trip)
  [GBxy] -> Output/2(GBxyin)
  [Trip] -> Excitation System/2(Trip)
  Output/1(m) -> m/1
  Mechanical DE/1(delta) -> Scope/1, "Machine Equations "/1(delta), [delta]
  Bistable2/2 -> Terminator/1
  [f] -> Output/5(fin)
  Output/2(Igxy1) -> Igxy1/1
  PSS1/1(Upss) -> Excitation System/1(Upss), Scope2/1
  "Machine Equations "/3(GBxy) -> Switch4/3
  Vgxy/1 -> "Machine Equations "/2(Vgxy)
  Constant/1 -> Switch4/1
  "Machine Equations "/2(Igxy1) -> pu->pu/1
  Governor/1(dPm) -> Mechanical DE/2(dPm), Scope3/1
  [delta] -> Output/3(deltain)
  [Vg] -> Output/6(Vg)
  [Igxy1] -> Output/1(Igxy1in)
  Mechanical DE/2(w) -> Governor/1(w), PSS1/1(w), [f]
  Output/3(GBxy) -> GBxy/1
  Excitation System/1(Ef) -> Scope5/1, "Machine Equations "/3(Ef)
  "Machine Equations "/4(Vg) -> [Vg], Excitation System/3(Vg)
  [Trip] -> "Machine Equations "/4(Trip)
  [Trip] -> Switch4/2
  Bistable2/1 -> [Trip]
  "Machine Equations "/1(Pe) -> Scope1/1, Mechanical DE/1(Pe), [Pe]
  [Pe] -> Output/4(Pein)
  Switch4/1 -> Gain1/1
  Trip/1 -> Bistable2/1
  Ground/1 -> Bistable2/2
  [Trip] -> Mechanical DE/3(Trip)

== system Two_area_system_with_wind_farm-DESKTOP-8DA4B7M/Network1 ==
  Ixy : Inport
  Clock : Clock
  Mux : Mux  Inputs=2
  S-Function : S-Function  FunctionName=TS_net_1_new  Parameters=busdata,linedata,VSS0,LINE,fbus,ng,Currentin_idx  SFunctionDeploymentMode=off  EnableBusSupport=off
  Vxy : Outport
  wires:
  Clock/1 -> Mux/1
  Ixy/1 -> Mux/2
  Mux/1 -> S-Function/1
  S-Function/1 -> Vxy/1

== system Two_area_system_with_wind_farm-DESKTOP-8DA4B7M/Network2 ==
  Ixy : Inport
  Clock : Clock
  Mux : Mux  Inputs=2
  S-Function : S-Function  FunctionName=TS_net_2_new  Parameters=busdata,linedata,VSS0,LINE,fbus,ng,Currentin_idx  SFunctionDeploymentMode=off  EnableBusSupport=off
  Vxy : Outport
  wires:
  Clock/1 -> Mux/1
  Ixy/1 -> Mux/2
  Mux/1 -> S-Function/1
  S-Function/1 -> Vxy/1

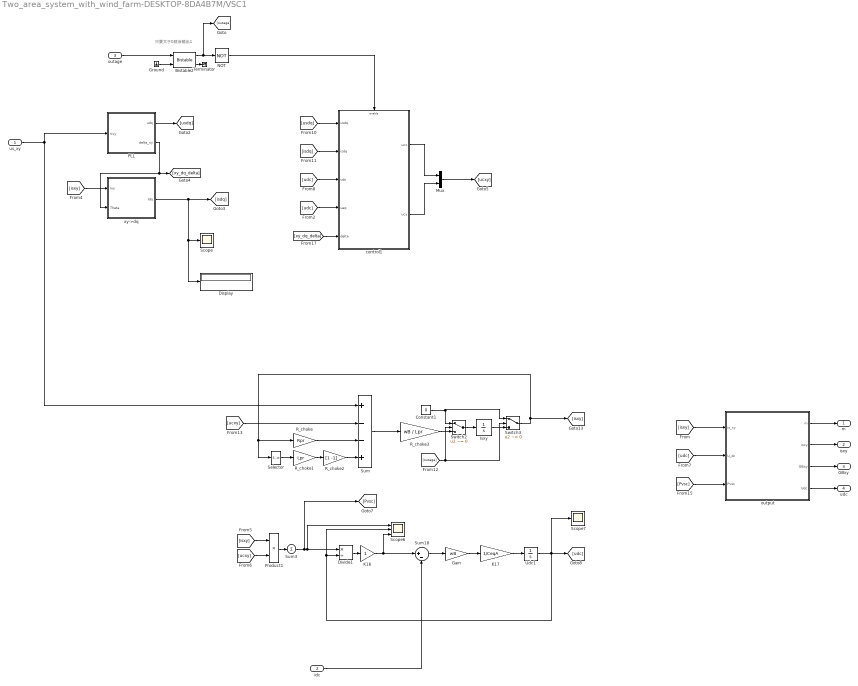
== system Two_area_system_with_wind_farm-DESKTOP-8DA4B7M/VSC1 ==
  note: 只要大于0就会输出1
  us_xy : Inport
  idc : Inport  Port=2
  outage : Inport  Port=3
  " control1" : Subsystem
  Bistable2 : powerlib_meascontrol/Logic/Bistable  Qpriority=Set  ic=0  Ts=0
      settings: SourceProductBaseCode=PS
  Constant1 : Constant  Value=0
  Display : Display
  Divide1 : Product  Inputs=*/
  Gain : Gain  Gain=wB
  Ground : Ground
  Isxy : Integrator  InitialCondition=[Is_xA_0 Is_yA_0]
  K16 : Gain  SaturateOnIntegerOverflow=on  OutDataTypeStr=Inherit: Same as input  ParamDataTypeStr=Inherit: Same as input
  K17 : Gain  Gain=1/CeqA  SaturateOnIntegerOverflow=on  OutDataTypeStr=Inherit: Same as input  ParamDataTypeStr=Inherit: Same as input
  Mux : Mux  Inputs=2
  NOT : Logic  Operator=NOT  AllPortsSameDT=off  OutDataTypeStr=boolean
  PLL : Subsystem  VariantControl=NoIdeal_PLL_VSC1
  Product1 : Product  Inputs=**  RndMeth=Zero
  R_choke : Gain  Gain=Rpr  SaturateOnIntegerOverflow=on  OutDataTypeStr=Inherit: Same as input  ParamDataTypeStr=Inherit: Same as input
  R_choke1 : Gain  Gain=Lpr  SaturateOnIntegerOverflow=on  OutDataTypeStr=Inherit: Same as input  ParamDataTypeStr=Inherit: Same as input
  R_choke2 : Gain  Gain=[1 -1]  SaturateOnIntegerOverflow=on  OutDataTypeStr=Inherit: Same as input  ParamDataTypeStr=Inherit: Same as input
  R_choke3 : Gain  Gain=wB / Lpr  SaturateOnIntegerOverflow=on  OutDataTypeStr=Inherit: Same as input  ParamDataTypeStr=Inherit: Same as input
  Scope : Scope
  Scope6 : Scope  NumInputPorts=3
  Scope7 : Scope
  Selector : Selector  InputPortWidth=2  IndexOptions=Index vector (dialog)  Indices=[2 1]  OutputSizes=1
  Sum : Sum  Inputs=+--+  SaturateOnIntegerOverflow=on
  Sum18 : Sum  Inputs=|+-  SaturateOnIntegerOverflow=on
  Sum3 : Sum  Inputs=1  InputSameDT=on  SaturateOnIntegerOverflow=on  OutDataTypeStr=Inherit: Same as first input
  Switch2 : Switch  Criteria=u2 ~= 0  Threshold=0.5  SaturateOnIntegerOverflow=on
  Switch3 : Switch  Criteria=u2 ~= 0  Threshold=0.5  SaturateOnIntegerOverflow=on
  Terminator : Terminator
  Udc1 : Integrator  InitialCondition=UeqA  UpperSaturationLimit=2  LowerSaturationLimit=-2
  output : Subsystem
  xy->dq : Subsystem
  m : Outport
  isxy : Outport  Port=2
  GBxy : Outport  Port=3
  udc : Outport  Port=4
  wires:
  Selector/1 -> R_choke1/1
  [Pvsc] -> output/3(Pvsc)
  Sum18/1 -> Gain/1
  Sum/1 -> R_choke3/1
  Gain/1 -> K17/1
  R_choke3/1 -> Switch2/3
  Divide1/1 -> K16/1
  [udc] -> output/2(U_dc)
  Ground/1 -> Bistable2/2
  R_choke2/1 -> Sum/4
  output/4(Udc) -> udc/1
  R_choke/1 -> Sum/3
  [ucxy] -> Sum/2
  idc/1 -> Sum18/2
  Product1/1 -> Sum3/1
  [isxy] -> Product1/1
  K17/1 -> Udc1/1
  us_xy/1 -> PLL/1(Vxy), Sum/1
  PLL/1(udq) -> [usdq]
  output/1(m) -> m/1
  Udc1/1 -> Scope7/1, [udc], Divide1/2, Scope6/2
  NOT/1 -> " control1"/Enable
  R_choke1/1 -> R_choke2/1
  Sum3/1 -> Divide1/1, Scope6/1, [Pvsc]
  [ucxy] -> Product1/2
  Bistable2/1 -> NOT/1, [outage]
  Isxy/1 -> Switch3/3
  [udc] -> " control1"/3(udc)
  PLL/2(delta_xy) -> [xy_dq_delta], xy->dq/2(Theta)
  [isxy] -> xy->dq/1(Ixy)
  [isxy] -> output/1(is_xy)
  output/2(isxy) -> isxy/1
  [xy_dq_delta] -> " control1"/5(delta)
  xy->dq/1(Idq) -> [isdq], Scope/1, Display/1
  Bistable2/2 -> Terminator/1
  outage/1 -> Bistable2/1
  [outage] -> Switch2/2, Switch3/2
  [isdq] -> " control1"/2(isdq)
  " control1"/1(ucx) -> Mux/1
  Switch2/1 -> Isxy/1
  Switch3/1 -> R_choke/1, Selector/1, [isxy]
  Mux/1 -> [ucxy]
  [udc] -> " control1"/4(ueq)
  [usdq] -> " control1"/1(usdq)
  K16/1 -> Scope6/3, Sum18/1
  output/3(GBxy) -> GBxy/1
  Constant1/1 -> Switch2/1, Switch3/1
  " control1"/2(ucy) -> Mux/2

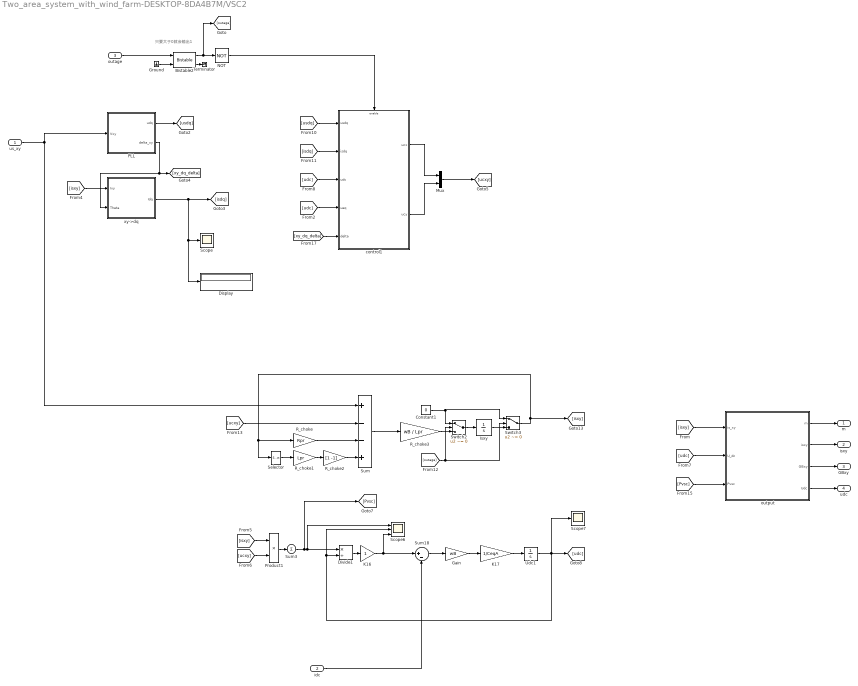
== system Two_area_system_with_wind_farm-DESKTOP-8DA4B7M/VSC2 ==
  note: 只要大于0就会输出1
  us_xy : Inport
  idc : Inport  Port=2
  outage : Inport  Port=3
  " control1" : Subsystem
  Bistable2 : powerlib_meascontrol/Logic/Bistable  Qpriority=Set  ic=0  Ts=0
      settings: SourceProductBaseCode=PS
  Constant1 : Constant  Value=0
  Display : Display
  Divide1 : Product  Inputs=*/
  Gain : Gain  Gain=wB
  Ground : Ground
  Isxy : Integrator  InitialCondition=[Is_xA_0 Is_yA_0]
  K16 : Gain  SaturateOnIntegerOverflow=on  OutDataTypeStr=Inherit: Same as input  ParamDataTypeStr=Inherit: Same as input
  K17 : Gain  Gain=1/CeqA  SaturateOnIntegerOverflow=on  OutDataTypeStr=Inherit: Same as input  ParamDataTypeStr=Inherit: Same as input
  Mux : Mux  Inputs=2
  NOT : Logic  Operator=NOT  AllPortsSameDT=off  OutDataTypeStr=boolean
  PLL : Subsystem  VariantControl=NoIdeal_PLL_VSC1
  Product1 : Product  Inputs=**  RndMeth=Zero
  R_choke : Gain  Gain=Rpr  SaturateOnIntegerOverflow=on  OutDataTypeStr=Inherit: Same as input  ParamDataTypeStr=Inherit: Same as input
  R_choke1 : Gain  Gain=Lpr  SaturateOnIntegerOverflow=on  OutDataTypeStr=Inherit: Same as input  ParamDataTypeStr=Inherit: Same as input
  R_choke2 : Gain  Gain=[1 -1]  SaturateOnIntegerOverflow=on  OutDataTypeStr=Inherit: Same as input  ParamDataTypeStr=Inherit: Same as input
  R_choke3 : Gain  Gain=wB / Lpr  SaturateOnIntegerOverflow=on  OutDataTypeStr=Inherit: Same as input  ParamDataTypeStr=Inherit: Same as input
  Scope : Scope
  Scope6 : Scope  NumInputPorts=3
  Scope7 : Scope
  Selector : Selector  InputPortWidth=2  IndexOptions=Index vector (dialog)  Indices=[2 1]  OutputSizes=1
  Sum : Sum  Inputs=+--+  SaturateOnIntegerOverflow=on
  Sum18 : Sum  Inputs=|+-  SaturateOnIntegerOverflow=on
  Sum3 : Sum  Inputs=1  InputSameDT=on  SaturateOnIntegerOverflow=on  OutDataTypeStr=Inherit: Same as first input
  Switch2 : Switch  Criteria=u2 ~= 0  Threshold=0.5  SaturateOnIntegerOverflow=on
  Switch3 : Switch  Criteria=u2 ~= 0  Threshold=0.5  SaturateOnIntegerOverflow=on
  Terminator : Terminator
  Udc1 : Integrator  InitialCondition=UeqA  UpperSaturationLimit=2  LowerSaturationLimit=-2
  output : Subsystem
  xy->dq : Subsystem
  m : Outport
  isxy : Outport  Port=2
  GBxy : Outport  Port=3
  udc : Outport  Port=4
  wires:
  Selector/1 -> R_choke1/1
  [Pvsc] -> output/3(Pvsc)
  Sum18/1 -> Gain/1
  Sum/1 -> R_choke3/1
  Gain/1 -> K17/1
  R_choke3/1 -> Switch2/3
  Divide1/1 -> K16/1
  [udc] -> output/2(U_dc)
  Ground/1 -> Bistable2/2
  R_choke2/1 -> Sum/4
  output/4(Udc) -> udc/1
  R_choke/1 -> Sum/3
  [ucxy] -> Sum/2
  idc/1 -> Sum18/2
  Product1/1 -> Sum3/1
  [isxy] -> Product1/1
  K17/1 -> Udc1/1
  us_xy/1 -> PLL/1(Vxy), Sum/1
  PLL/1(udq) -> [usdq]
  output/1(m) -> m/1
  Udc1/1 -> Scope7/1, [udc], Divide1/2, Scope6/2
  NOT/1 -> " control1"/Enable
  R_choke1/1 -> R_choke2/1
  Sum3/1 -> Divide1/1, Scope6/1, [Pvsc]
  [ucxy] -> Product1/2
  Bistable2/1 -> NOT/1, [outage]
  Isxy/1 -> Switch3/3
  [udc] -> " control1"/3(udc)
  PLL/2(delta_xy) -> [xy_dq_delta], xy->dq/2(Theta)
  [isxy] -> xy->dq/1(Ixy)
  [isxy] -> output/1(is_xy)
  output/2(isxy) -> isxy/1
  [xy_dq_delta] -> " control1"/5(delta)
  xy->dq/1(Idq) -> [isdq], Scope/1, Display/1
  Bistable2/2 -> Terminator/1
  outage/1 -> Bistable2/1
  [outage] -> Switch2/2, Switch3/2
  [isdq] -> " control1"/2(isdq)
  " control1"/1(ucx) -> Mux/1
  Switch2/1 -> Isxy/1
  Switch3/1 -> R_choke/1, Selector/1, [isxy]
  Mux/1 -> [ucxy]
  [udc] -> " control1"/4(ueq)
  [usdq] -> " control1"/1(usdq)
  K16/1 -> Scope6/3, Sum18/1
  output/3(GBxy) -> GBxy/1
  Constant1/1 -> Switch2/1, Switch3/1
  " control1"/2(ucy) -> Mux/2

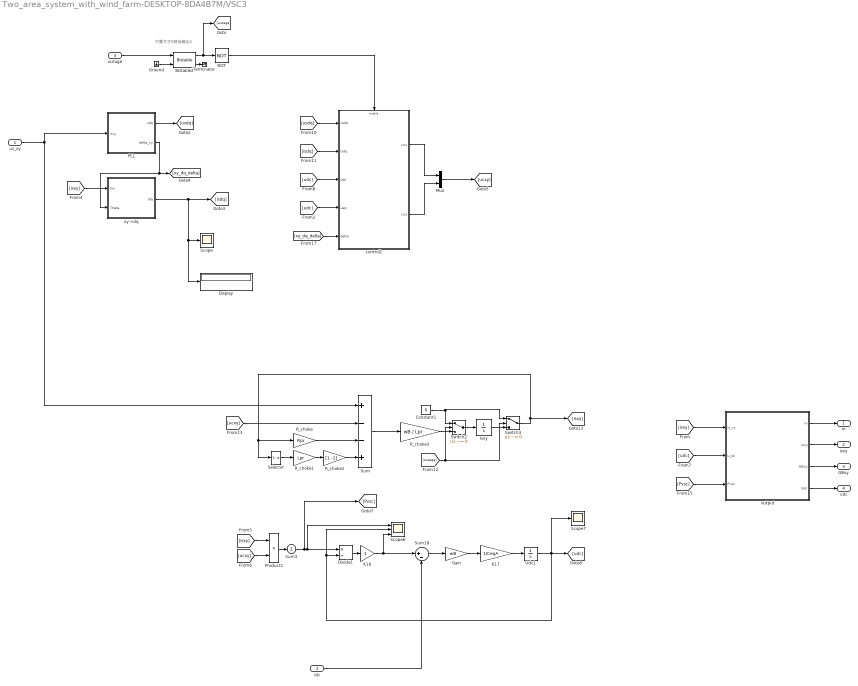
== system Two_area_system_with_wind_farm-DESKTOP-8DA4B7M/VSC3 ==
  note: 只要大于0就会输出1
  us_xy : Inport
  idc : Inport  Port=2
  outage : Inport  Port=3
  " control1" : Subsystem
  Bistable2 : powerlib_meascontrol/Logic/Bistable  Qpriority=Set  ic=0  Ts=0
      settings: SourceProductBaseCode=PS
  Constant1 : Constant  Value=0
  Display : Display
  Divide1 : Product  Inputs=*/
  Gain : Gain  Gain=wB
  Ground : Ground
  Isxy : Integrator  InitialCondition=[Is_xA_0 Is_yA_0]
  K16 : Gain  SaturateOnIntegerOverflow=on  OutDataTypeStr=Inherit: Same as input  ParamDataTypeStr=Inherit: Same as input
  K17 : Gain  Gain=1/CeqA  SaturateOnIntegerOverflow=on  OutDataTypeStr=Inherit: Same as input  ParamDataTypeStr=Inherit: Same as input
  Mux : Mux  Inputs=2
  NOT : Logic  Operator=NOT  AllPortsSameDT=off  OutDataTypeStr=boolean
  PLL : Subsystem  VariantControl=NoIdeal_PLL_VSC1
  Product1 : Product  Inputs=**  RndMeth=Zero
  R_choke : Gain  Gain=Rpr  SaturateOnIntegerOverflow=on  OutDataTypeStr=Inherit: Same as input  ParamDataTypeStr=Inherit: Same as input
  R_choke1 : Gain  Gain=Lpr  SaturateOnIntegerOverflow=on  OutDataTypeStr=Inherit: Same as input  ParamDataTypeStr=Inherit: Same as input
  R_choke2 : Gain  Gain=[1 -1]  SaturateOnIntegerOverflow=on  OutDataTypeStr=Inherit: Same as input  ParamDataTypeStr=Inherit: Same as input
  R_choke3 : Gain  Gain=wB / Lpr  SaturateOnIntegerOverflow=on  OutDataTypeStr=Inherit: Same as input  ParamDataTypeStr=Inherit: Same as input
  Scope : Scope
  Scope6 : Scope  NumInputPorts=3
  Scope7 : Scope
  Selector : Selector  InputPortWidth=2  IndexOptions=Index vector (dialog)  Indices=[2 1]  OutputSizes=1
  Sum : Sum  Inputs=+--+  SaturateOnIntegerOverflow=on
  Sum18 : Sum  Inputs=|+-  SaturateOnIntegerOverflow=on
  Sum3 : Sum  Inputs=1  InputSameDT=on  SaturateOnIntegerOverflow=on  OutDataTypeStr=Inherit: Same as first input
  Switch2 : Switch  Criteria=u2 ~= 0  Threshold=0.5  SaturateOnIntegerOverflow=on
  Switch3 : Switch  Criteria=u2 ~= 0  Threshold=0.5  SaturateOnIntegerOverflow=on
  Terminator : Terminator
  Udc1 : Integrator  InitialCondition=UeqA  UpperSaturationLimit=2  LowerSaturationLimit=-2
  output : Subsystem
  xy->dq : Subsystem
  m : Outport
  isxy : Outport  Port=2
  GBxy : Outport  Port=3
  udc : Outport  Port=4
  wires:
  Selector/1 -> R_choke1/1
  [Pvsc] -> output/3(Pvsc)
  Sum18/1 -> Gain/1
  Sum/1 -> R_choke3/1
  Gain/1 -> K17/1
  R_choke3/1 -> Switch2/3
  Divide1/1 -> K16/1
  [udc] -> output/2(U_dc)
  Ground/1 -> Bistable2/2
  R_choke2/1 -> Sum/4
  output/4(Udc) -> udc/1
  R_choke/1 -> Sum/3
  [ucxy] -> Sum/2
  idc/1 -> Sum18/2
  Product1/1 -> Sum3/1
  [isxy] -> Product1/1
  K17/1 -> Udc1/1
  us_xy/1 -> PLL/1(Vxy), Sum/1
  PLL/1(udq) -> [usdq]
  output/1(m) -> m/1
  Udc1/1 -> Scope7/1, [udc], Divide1/2, Scope6/2
  NOT/1 -> " control1"/Enable
  R_choke1/1 -> R_choke2/1
  Sum3/1 -> Divide1/1, Scope6/1, [Pvsc]
  [ucxy] -> Product1/2
  Bistable2/1 -> NOT/1, [outage]
  Isxy/1 -> Switch3/3
  [udc] -> " control1"/3(udc)
  PLL/2(delta_xy) -> [xy_dq_delta], xy->dq/2(Theta)
  [isxy] -> xy->dq/1(Ixy)
  [isxy] -> output/1(is_xy)
  output/2(isxy) -> isxy/1
  [xy_dq_delta] -> " control1"/5(delta)
  xy->dq/1(Idq) -> [isdq], Scope/1, Display/1
  Bistable2/2 -> Terminator/1
  outage/1 -> Bistable2/1
  [outage] -> Switch2/2, Switch3/2
  [isdq] -> " control1"/2(isdq)
  " control1"/1(ucx) -> Mux/1
  Switch2/1 -> Isxy/1
  Switch3/1 -> R_choke/1, Selector/1, [isxy]
  Mux/1 -> [ucxy]
  [udc] -> " control1"/4(ueq)
  [usdq] -> " control1"/1(usdq)
  K16/1 -> Scope6/3, Sum18/1
  output/3(GBxy) -> GBxy/1
  Constant1/1 -> Switch2/1, Switch3/1
  " control1"/2(ucy) -> Mux/2
